simulink model "lab10_compare_sl"  (R2021b)
settings: Solver=VariableStepAuto  StartTime=0.0  StopTime=150.0  RelTol=1e-3
libraries: simulink x2
settings Model: Creator=JaSzw  LastModifiedBy=JaSzw

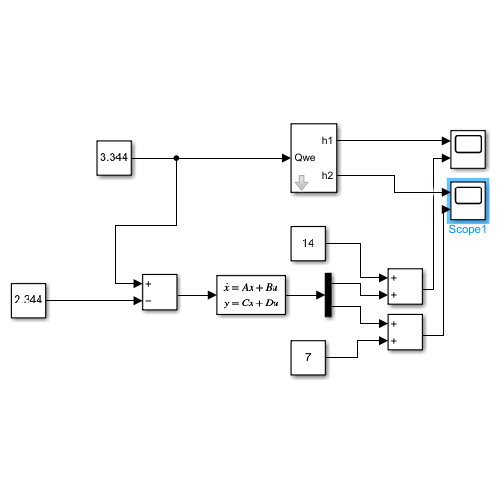
[thumbnail: Simulink's stored preview of the top-level diagram]
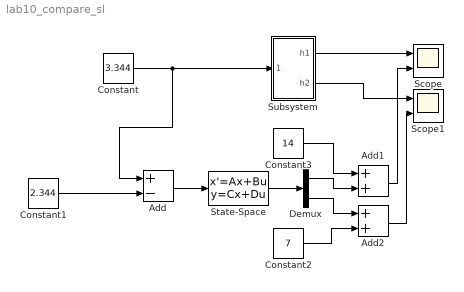
== system lab10_compare_sl ==
  Add : Sum  Inputs=+-
  Add1 : Sum
  Add2 : Sum
  Constant : Constant  Value=3.344
  Constant1 : Constant  Value=2.344
  Constant2 : Constant  Value=7
  Constant3 : Constant  Value=14
  Demux : Demux  Outputs=2
  Scope : Scope  NumInputPorts=2
  Scope1 : Scope  NumInputPorts=2
  State-Space : StateSpace  A=[-0.167417357020601,0.167417357013755;0.083708678510301,-0.167417357013755]  B=[1;0]  C=[1,0;0,1]  D=[0;0]  InitialCondition=[-10;-5]
  Subsystem : Subsystem  mask{h1=4, h2=2, S1=1, S2=2, Swy1=0.2, Swy2=0.2, fi1=1, fi2=1, g=9.81, Qwe=2}
  wires:
  Add/1 -> State-Space/1
  Add1/1 -> Scope/2
  Demux/2 -> Add2/1
  Demux/1 -> Add1/2
  Constant2/1 -> Add2/2
  State-Space/1 -> Demux/1
  Constant1/1 -> Add/2
  Constant3/1 -> Add1/1
  Constant/1 -> Add/1, Subsystem/1(Qwe)
  Subsystem/2(h2) -> Scope1/1
  Add2/1 -> Scope1/2
  Subsystem/1(h1) -> Scope/1

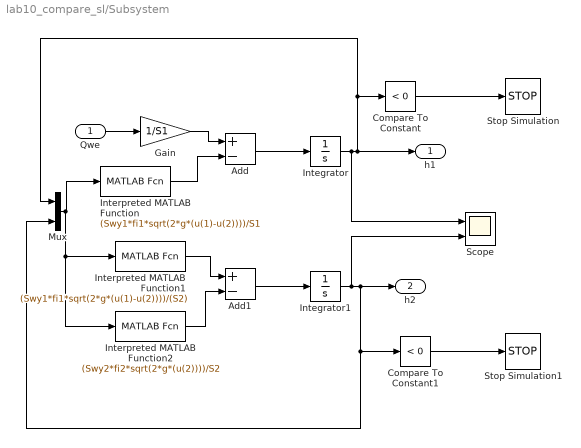
== system lab10_compare_sl/Subsystem ==
  Qwe : Inport
  Add : Sum  Inputs=+-
  Add1 : Sum  Inputs=+-
  Compare To Constant : simulink/Logic and Bit Operations/Compare To Constant  relop=<  const=0  OutDataTypeStr=boolean
  Compare To Constant1 : simulink/Logic and Bit Operations/Compare To Constant  relop=<  const=0  OutDataTypeStr=boolean
  Gain : Gain  Gain=1/S1
  Integrator : Integrator  InitialCondition=h1
  Integrator1 : Integrator  InitialCondition=h2
  Interpreted MATLAB Function : MATLABFcn  MATLABFcn=(Swy1*fi1*sqrt(2*g*(u(1)-u(2))))/S1  OutputDimensions=1
  Interpreted MATLAB Function1 : MATLABFcn  MATLABFcn=(Swy1*fi1*sqrt(2*g*(u(1)-u(2))))/(S2)  OutputDimensions=1
  Interpreted MATLAB Function2 : MATLABFcn  MATLABFcn=(Swy2*fi2*sqrt(2*g*(u(2))))/S2  OutputDimensions=1
  Mux : Mux  Inputs=2
  Scope : Scope  NumInputPorts=2
  Stop Simulation : Stop
  Stop Simulation1 : Stop
  h1 : Outport
  h2 : Outport  Port=2
  wires:
  Integrator/1 -> Scope/1, h1/1, Compare To Constant/1, Mux/1
  Add1/1 -> Integrator1/1
  Add/1 -> Integrator/1
  Interpreted MATLAB Function/1 -> Add/2
  Qwe/1 -> Gain/1
  Mux/1 -> Interpreted MATLAB Function2/1, Interpreted MATLAB Function1/1, Interpreted MATLAB Function/1
  Interpreted MATLAB Function2/1 -> Add1/2
  Interpreted MATLAB Function1/1 -> Add1/1
  Compare To Constant/1 -> Stop Simulation/1
  Integrator1/1 -> Scope/2, h2/1, Compare To Constant1/1, Mux/2
  Compare To Constant1/1 -> Stop Simulation1/1
  Gain/1 -> Add/1
